simulink model "covid_lineal_unforced"  (R2023a)
settings: Solver=VariableStepAuto  StartTime=0.0  StopTime=365  RelTol=1e-3
values from neighbouring files (symbols this model uses):
  A = [-0.00502784 -1.6e-07 0 2.8e-05 0 0 0 0.005 0 -0.166666666667 0 0 ... (64 elements, 8x8)]    [matrices.mat]
  B = [-1 0 0 0 0 0 0 1]    [matrices.mat]
  C = [1 0 0 0 0 0 0 0 0 1 0 0 ... (64 elements, 8x8)]    [matrices.mat]
  N = 7500000    [parameters_covid.mat]
  vector_constants = [-1.6e-07 1.6e-07 0 0 0 0 0 0]    [matrices.mat]
settings Model: Creator=User  LastModifiedBy=mluser

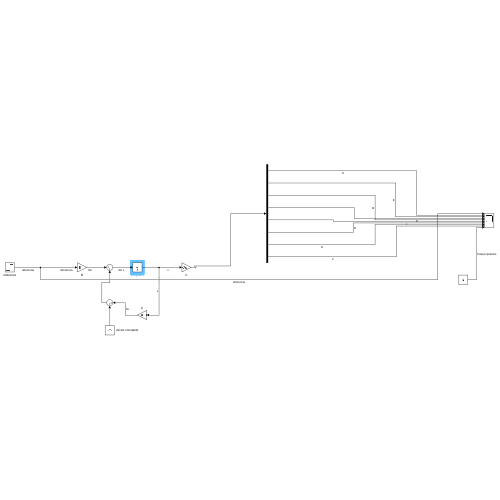
[thumbnail: Simulink's stored preview of the top-level diagram]
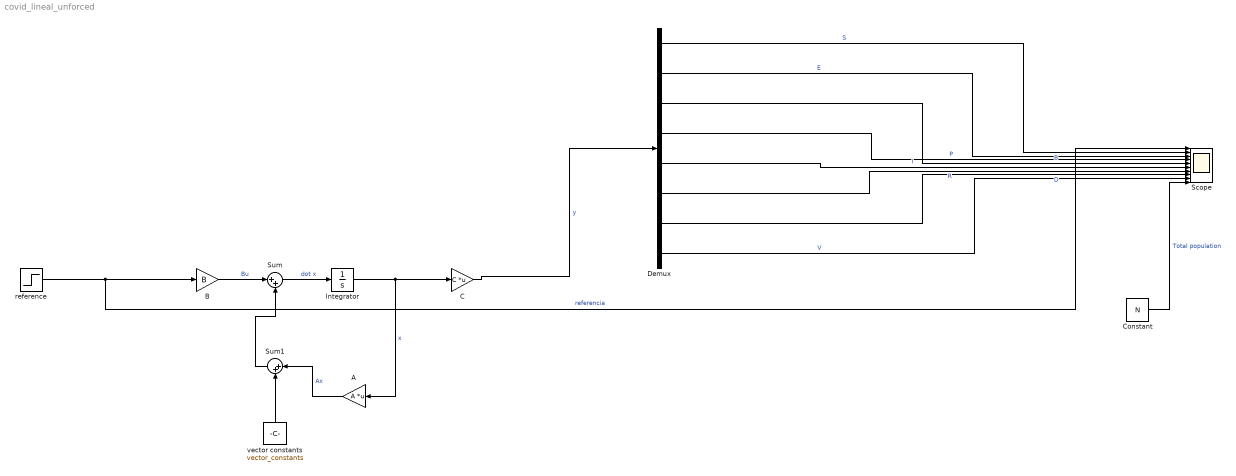
== system covid_lineal_unforced ==
  A : Gain  Gain=A  Multiplication=Matrix(K*u)
  B : Gain  Gain=B
  C : Gain  Gain=C  Multiplication=Matrix(K*u)
  Constant : Constant  Value=N
  Demux : Demux  Outputs=8
  Integrator : Integrator  InitialCondition=[N*0.85; N*0.05;0;0;N*0.1;0;0;0]
  Scope : Scope  NumInputPorts=10
  Sum : Sum  Inputs=|++
  Sum1 : Sum  Inputs=|++
  reference : Step  SampleTime=0
  vector constants : Constant  Value=vector_constants
  wires:
  Integrator/1 -> A/1, C/1  "x"
  B/1 -> Sum/1  "Bu"
  Sum/1 -> Integrator/1  "dot x"
  reference/1 -> Scope/1, B/1  "referencia"
  A/1 -> Sum1/1  "Ax"
  Sum1/1 -> Sum/2
  C/1 -> Demux/1  "y"
  Demux/1 -> Scope/2  "S"
  Demux/2 -> Scope/3  "E"
  Demux/3 -> Scope/5  "B"
  Demux/4 -> Scope/4  "P"
  Demux/5 -> Scope/6  "I"
  Demux/6 -> Scope/7  "R"
  Demux/7 -> Scope/8  "D"
  Demux/8 -> Scope/9  "V"
  vector constants/1 -> Sum1/2
  Constant/1 -> Scope/10  "Total population"
